simulink model "TwoTankSystem_Linearize"  (R2013b)
settings: Solver=ode4  StartTime=0.0  StopTime=SIM_TIME  FixedStep=STEP_SIZE  RelTol=1e-3
undefined symbols (not defined in the file): At, C0, Dv, ka, kh, kt, x0
settings Model: Creator=roga  LastModifiedBy=roga
settings DataIOCC: SaveFinalState=on
settings DebuggingCC: StateNameClashWarn=warning

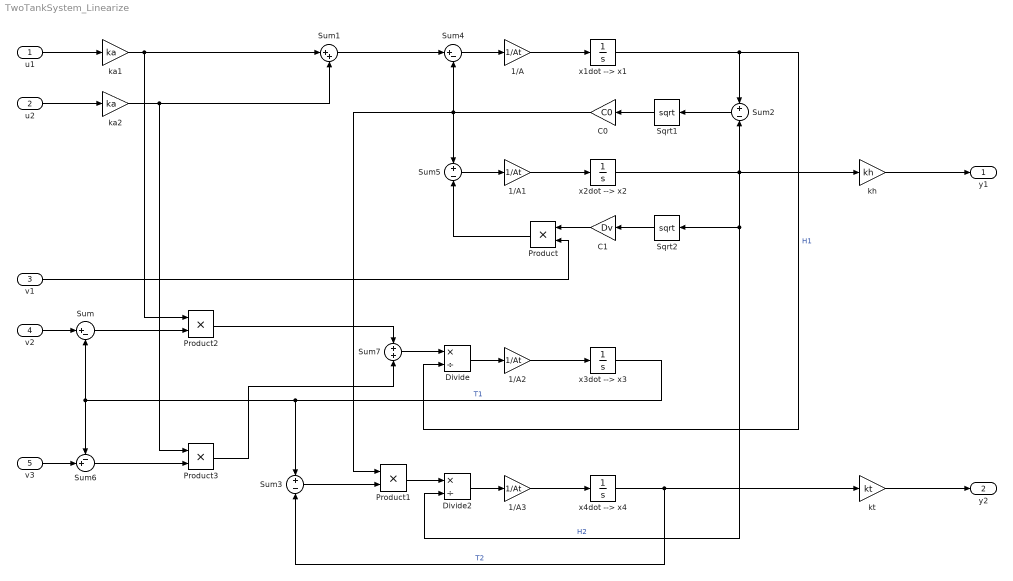
== system TwoTankSystem_Linearize ==
  u1 : Inport
  u2 : Inport  Port=2
  v1 : Inport  Port=3
  v2 : Inport  Port=4
  v3 : Inport  Port=5
  1/A{,1..3} (4 alike) : Gain  Gain=1/At
  C0 : Gain  Gain=C0
  C1 : Gain  Gain=Dv
  Divide : Product  Inputs=*/
  Divide2 : Product  Inputs=*/
  Product{,1..3} (4 alike) : Product
  Sqrt1 : Sqrt  SaturateOnIntegerOverflow=on
  Sqrt2 : Sqrt  SaturateOnIntegerOverflow=on
  Sum : Sum  Inputs=|+-
  Sum1 : Sum  Inputs=|++
  Sum2 : Sum  Inputs=+-
  Sum3 : Sum  Inputs=+-
  Sum4 : Sum  Inputs=|+-
  Sum5 : Sum  Inputs=+-
  Sum6 : Sum  Inputs=-+|
  Sum7 : Sum
  ka1 : Gain  Gain=ka
  ka2 : Gain  Gain=ka
  kh : Gain  Gain=kh
  kt : Gain  Gain=kt
  x1dot --> x1 : Integrator  Priority=1  InitialCondition=x0(1)  LimitOutput=on  LowerSaturationLimit=0
  x2dot --> x2 : Integrator  Priority=2  InitialCondition=x0(2)  LimitOutput=on  LowerSaturationLimit=0
  x3dot --> x3 : Integrator  Priority=3  InitialCondition=x0(3)
  x4dot --> x4 : Integrator  Priority=4  InitialCondition=x0(4)
  y1 : Outport
  y2 : Outport  Port=2
  wires:
  Product1/1 -> Divide2/1
  Divide/1 -> 1/A2/1
  Sum6/1 -> Product3/2
  1/A1/1 -> x2dot --> x2/1
  Sum5/1 -> 1/A1/1
  Product/1 -> Sum5/2
  x1dot --> x1/1 -> Sum2/1, Divide/2  "H1"
  Sum/1 -> Product2/2
  C1/1 -> Product/1
  Sum3/1 -> Product1/2
  Sqrt2/1 -> C1/1
  1/A2/1 -> x3dot --> x3/1
  x4dot --> x4/1 -> kt/1, Sum3/2  "T2"
  C0/1 -> Sum4/2, Product1/1, Sum5/1
  1/A3/1 -> x4dot --> x4/1
  x2dot --> x2/1 -> kh/1, Divide2/2, Sqrt2/1, Sum2/2  "H2"
  Divide2/1 -> 1/A3/1
  Sum7/1 -> Divide/1
  Product2/1 -> Sum7/1
  ka1/1 -> Product2/1, Sum1/1
  Product3/1 -> Sum7/2
  ka2/1 -> Product3/1, Sum1/2
  x3dot --> x3/1 -> Sum3/1, Sum6/1, Sum/2  "T1"
  1/A/1 -> x1dot --> x1/1
  Sum1/1 -> Sum4/1
  Sqrt1/1 -> C0/1
  Sum4/1 -> 1/A/1
  Sum2/1 -> Sqrt1/1
  v1/1 -> Product/2
  v2/1 -> Sum/1
  v3/1 -> Sum6/2
  u1/1 -> ka1/1
  u2/1 -> ka2/1
  kh/1 -> y1/1
  kt/1 -> y2/1
